simulink model "flightsim_simple_ode_3D_1_5_ListedAssumptions"  (R2020b)
settings: Solver=VariableStepAuto  StartTime=0.0  StopTime=12  RelTol=1e-3
libraries: simulink x3, pid_lib x2
settings Model: Creator=jonathan  LastModifiedBy=jonathan

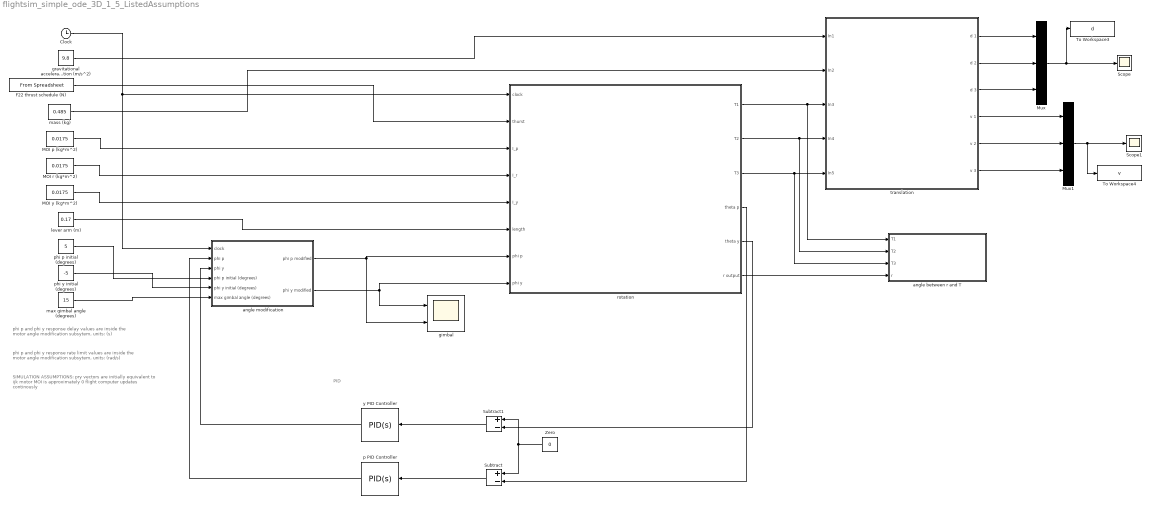
== system flightsim_simple_ode_3D_1_5_ListedAssumptions ==
  note: PID
  note: SIMULATION ASSUMPTIONS:
      | pry vectors are initially equivalent to ijk
      | motor MOI is approximately 0
      | flight computer updates continously
  note: phi p and phi y response rate limit values are inside the motor angle modification subsytem, units: (rad/s)
  note: phi p and phi y response delay values are inside the motor angle modification subsytem, units: (s)
  Clock : Clock
  F22 thrust schedule (N) : FromSpreadsheet  FileName=/Users/jonathan/Documents/GitHub/TVC-6DOF-Flight-Simulation/F15_thrust_curve.xlsx  OutDataTypeStr=double  ExtrapolationBeforeFirstDataPoint=Hold first value  ExtrapolationAfterLastDataPoint=Hold last value
  MOI p (kg*m^2) : Constant  Value=0.0175
  MOI r (kg*m^2) : Constant  Value=0.0175
  MOI y (kg*m^2) : Constant  Value=0.0175
  Mux : Mux  Inputs=3
  Mux1 : Mux  Inputs=3
  Scope : Scope
  Scope1 : Scope
  Subtract : Sum  Inputs=+-
  Subtract1 : Sum  Inputs=+-
  To Workspace3 : ToWorkspace  VariableName=d  SaveFormat=Timeseries  SampleTime=-1
  To Workspace4 : ToWorkspace  VariableName=v  SaveFormat=Timeseries  SampleTime=-1
  Zero : Constant  Value=0  OutDataTypeStr=Inherit: Inherit via back propagation
  angle between r and T : Subsystem
  angle modification : Subsystem
  gimbal : Scope  NumInputPorts=2
  gravitational acceleration (m/s^2) : Constant  Value=9.8
  lever arm (m) : Constant  Value=0.17
  mass (kg) : Constant  Value=0.485
  max gimbal angle (degrees) : Constant  Value=15
  p PID Controller : pid_lib/PID Controller  Controller=PID  Form=Parallel  TimeDomain=Continuous-time  UseExternalTs=off  SampleTime=-1  IntegratorMethod=Forward Euler  FilterMethod=Forward Euler  ControllerParametersSource=internal  P=-0.00942  I=-0.00055  D=-0.03588  UseFilter=on  N=1142.8279760416  TunerSelectOption=Transfer Function Based (PID Tuner App)  InitialConditionSource=internal  InitialConditionForIntegrator=0  InitialConditionForFilter=0  DifferentiatorICPrevScaledInput=0  ExternalReset=none  TrackingMode=off  Kt=1  LimitOutput=off  SatLimitsSource=internal  UpperSaturationLimit=inf  LowerSaturationLimit=-inf  LinearizeAsGain=on  AntiWindupMode=none  Kb=1  POutMin=[]  POutMax=[]  IOutMin=[]  IOutMax=[]  DOutMin=[]  DOutMax=[]  NOutMin=[]  NOutMax=[]  SumOutMin=[]  SumOutMax=[]  SaturationOutMin=[]  SaturationOutMax=[]  PParamMin=[]  PParamMax=[]  IParamMin=[]  IParamMax=[]  DParamMin=[]  DParamMax=[]  NParamMin=[]  NParamMax=[]  KbParamMin=[]  KbParamMax=[]  KtParamMin=[]  KtParamMax=[]  KbOutMin=[]  KbOutMax=[]  KtOutMin=[]  KtOutMax=[]  IntegratorOutMin=[]  IntegratorOutMax=[]  FilterOutMin=[]  FilterOutMax=[]  SumI1OutMin=[]  SumI1OutMax=[]  SumI2OutMin=[]  SumI2OutMax=[]  SumI3OutMin=[]  SumI3OutMax=[]  SumI4OutMin=[]  SumI4OutMax=[]  SumDOutMin=[]  SumDOutMax=[]  DifferentiatorOutMin=[]  DifferentiatorOutMax=[]  FilterDiffOutCoefMin=[]  FilterDiffOutCoefMax=[]  ReciprocalOutMin=[]  ReciprocalOutMax=[]  SumDenOutMin=[]  SumDenOutMax=[]  SumNumOutMin=[]  SumNumOutMax=[]  DivideOutMin=[]  DivideOutMax=[]  UdiffTsProdOutMin=[]  UdiffTsProdOutMax=[]  NTsProdOutMin=[]  NTsProdOutMax=[]  UintegralTsProdOutMin=[]  UintegralTsProdOutMax=[]  UngainTsProdOutMin=[]  UngainTsProdOutMax=[]  IntegratorContinuousStateAttributes=''  IntegratorStateMustResolveToSignalObject=off  IntegratorRTWStateStorageClass=Auto  FilterContinuousStateAttributes=''  FilterStateMustResolveToSignalObject=off  FilterRTWStateStorageClass=Auto  ParallelPVariant=InternalParameters  IdealPVariant=Disabled  IVariant=InternalParameters  DVariant=InternalParameters  IntegratorVariant=Continuous  SatVariant=Disabled  AWVariant=Passthrough  PCopyVariant=Disabled  TRVariant=Disabled  FdbkBlocksVariant=Forward  IdealPFdbkVariant=Disabled  SatFdbkVariant=Disabled  DerivativeFilterVariant=ContFilter  NVariant=InternalParameters  NCopyVariant=Disabled  FilterICVariant=InternalICsFilter  IntegratorICVariant=InternalICs  ExternalResetVariant=Disabled  TRSumVariant=Passthrough  SumFdbkVariant=Disabled  SumVariant=Sum_PID  TsampFilterVariant=InternalTs  TsampNgainVariant=Passthrough  TsampIntegralVariant=Passthrough  ExternalSaturationOutDataTypeStr=Inherit: Same as second input
  phi p initial (degrees) : Constant  Value=5
  phi y initial (degrees) : Constant  Value=-5
  rotation : Subsystem
  translation : Subsystem
  y PID Controller : pid_lib/PID Controller  Controller=PID  Form=Parallel  TimeDomain=Continuous-time  UseExternalTs=off  SampleTime=-1  IntegratorMethod=Forward Euler  FilterMethod=Forward Euler  ControllerParametersSource=internal  P=0.01930  I=0.00113  D=0.07350  UseFilter=on  N=1142.8279760416  TunerSelectOption=Transfer Function Based (PID Tuner App)  InitialConditionSource=internal  InitialConditionForIntegrator=0  InitialConditionForFilter=0  DifferentiatorICPrevScaledInput=0  ExternalReset=none  TrackingMode=off  Kt=1  LimitOutput=off  SatLimitsSource=internal  UpperSaturationLimit=inf  LowerSaturationLimit=-inf  LinearizeAsGain=on  AntiWindupMode=none  Kb=1  POutMin=[]  POutMax=[]  IOutMin=[]  IOutMax=[]  DOutMin=[]  DOutMax=[]  NOutMin=[]  NOutMax=[]  SumOutMin=[]  SumOutMax=[]  SaturationOutMin=[]  SaturationOutMax=[]  PParamMin=[]  PParamMax=[]  IParamMin=[]  IParamMax=[]  DParamMin=[]  DParamMax=[]  NParamMin=[]  NParamMax=[]  KbParamMin=[]  KbParamMax=[]  KtParamMin=[]  KtParamMax=[]  KbOutMin=[]  KbOutMax=[]  KtOutMin=[]  KtOutMax=[]  IntegratorOutMin=[]  IntegratorOutMax=[]  FilterOutMin=[]  FilterOutMax=[]  SumI1OutMin=[]  SumI1OutMax=[]  SumI2OutMin=[]  SumI2OutMax=[]  SumI3OutMin=[]  SumI3OutMax=[]  SumI4OutMin=[]  SumI4OutMax=[]  SumDOutMin=[]  SumDOutMax=[]  DifferentiatorOutMin=[]  DifferentiatorOutMax=[]  FilterDiffOutCoefMin=[]  FilterDiffOutCoefMax=[]  ReciprocalOutMin=[]  ReciprocalOutMax=[]  SumDenOutMin=[]  SumDenOutMax=[]  SumNumOutMin=[]  SumNumOutMax=[]  DivideOutMin=[]  DivideOutMax=[]  UdiffTsProdOutMin=[]  UdiffTsProdOutMax=[]  NTsProdOutMin=[]  NTsProdOutMax=[]  UintegralTsProdOutMin=[]  UintegralTsProdOutMax=[]  UngainTsProdOutMin=[]  UngainTsProdOutMax=[]  IntegratorContinuousStateAttributes=''  IntegratorStateMustResolveToSignalObject=off  IntegratorRTWStateStorageClass=Auto  FilterContinuousStateAttributes=''  FilterStateMustResolveToSignalObject=off  FilterRTWStateStorageClass=Auto  ParallelPVariant=InternalParameters  IdealPVariant=Disabled  IVariant=InternalParameters  DVariant=InternalParameters  IntegratorVariant=Continuous  SatVariant=Disabled  AWVariant=Passthrough  PCopyVariant=Disabled  TRVariant=Disabled  FdbkBlocksVariant=Forward  IdealPFdbkVariant=Disabled  SatFdbkVariant=Disabled  DerivativeFilterVariant=ContFilter  NVariant=InternalParameters  NCopyVariant=Disabled  FilterICVariant=InternalICsFilter  IntegratorICVariant=InternalICs  ExternalResetVariant=Disabled  TRSumVariant=Passthrough  SumFdbkVariant=Disabled  SumVariant=Sum_PID  TsampFilterVariant=InternalTs  TsampNgainVariant=Passthrough  TsampIntegralVariant=Passthrough  ExternalSaturationOutDataTypeStr=Inherit: Same as second input
  wires:
  MOI p (kg*m^2)/1 -> rotation/3(I_p)
  MOI r (kg*m^2)/1 -> rotation/4(I_r)
  MOI y (kg*m^2)/1 -> rotation/5(I_y)
  lever arm (m)/1 -> rotation/6(length)
  rotation/6(r output) -> angle between r and T/4(r)
  gravitational acceleration (m/s^2)/1 -> translation/1(In1)
  mass (kg)/1 -> translation/2(In2)
  rotation/1(T1) -> translation/3(In3), angle between r and T/1(T1)
  rotation/2(T2) -> translation/4(In4), angle between r and T/2(T2)
  rotation/3(T3) -> translation/5(In5), angle between r and T/3(T3)
  translation/4(v 1) -> Mux1/1
  translation/5(v 2) -> Mux1/2
  translation/6(v 3) -> Mux1/3
  translation/1(d 1) -> Mux/1
  translation/2(d 2) -> Mux/2
  translation/3(d 3) -> Mux/3
  Mux/1 -> To Workspace3/1, Scope/1
  Mux1/1 -> Scope1/1, To Workspace4/1
  F22 thrust schedule (N)/1 -> rotation/2(thurst)
  phi y initial (degrees)/1 -> angle modification/5(phi y initial (degrees))
  phi p initial (degrees)/1 -> angle modification/4(phi p initial (degrees))
  Clock/1 -> angle modification/1(clock), rotation/1(clock)
  y PID Controller/1 -> angle modification/3(phi y)
  p PID Controller/1 -> angle modification/2(phi p)
  angle modification/2(phi y modified) -> rotation/8(phi y), gimbal/1
  Zero/1 -> Subtract1/1, Subtract/1
  Subtract1/1 -> y PID Controller/1
  rotation/5(theta y) -> Subtract1/2
  rotation/4(theta p) -> Subtract/2
  angle modification/1(phi p modified) -> rotation/7(phi p), gimbal/2
  max gimbal angle (degrees)/1 -> angle modification/6(max gimbal angle (degrees))
  Subtract/1 -> p PID Controller/1

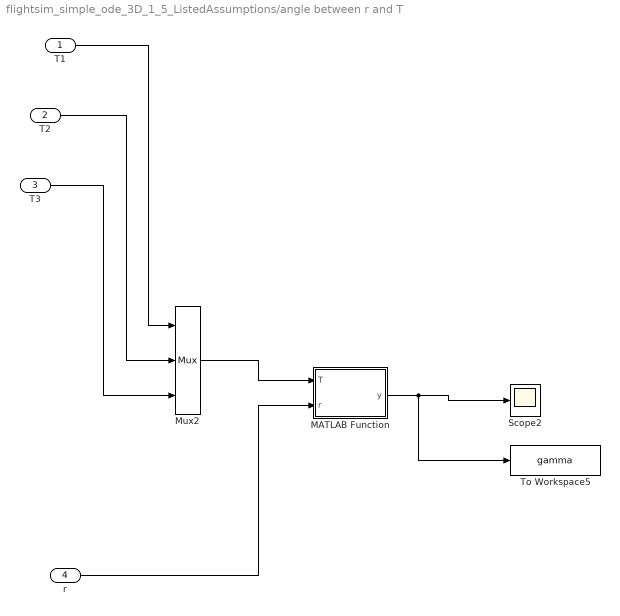
== system flightsim_simple_ode_3D_1_5_ListedAssumptions/angle between r and T ==
  T1 : Inport
  T2 : Inport  Port=2
  T3 : Inport  Port=3
  r : Inport  Port=4
  MATLAB Function : MATLAB Function  TreatAsAtomicUnit=on
  Mux2 : Mux  Inputs=3
  Scope2 : Scope
  To Workspace5 : ToWorkspace  VariableName=gamma  SaveFormat=Timeseries  SampleTime=-1
  wires:
  T3/1 -> Mux2/3
  r/1 -> MATLAB Function/2(r)
  T2/1 -> Mux2/2
  T1/1 -> Mux2/1
  Mux2/1 -> MATLAB Function/1(T)
  MATLAB Function/1(y) -> To Workspace5/1, Scope2/1

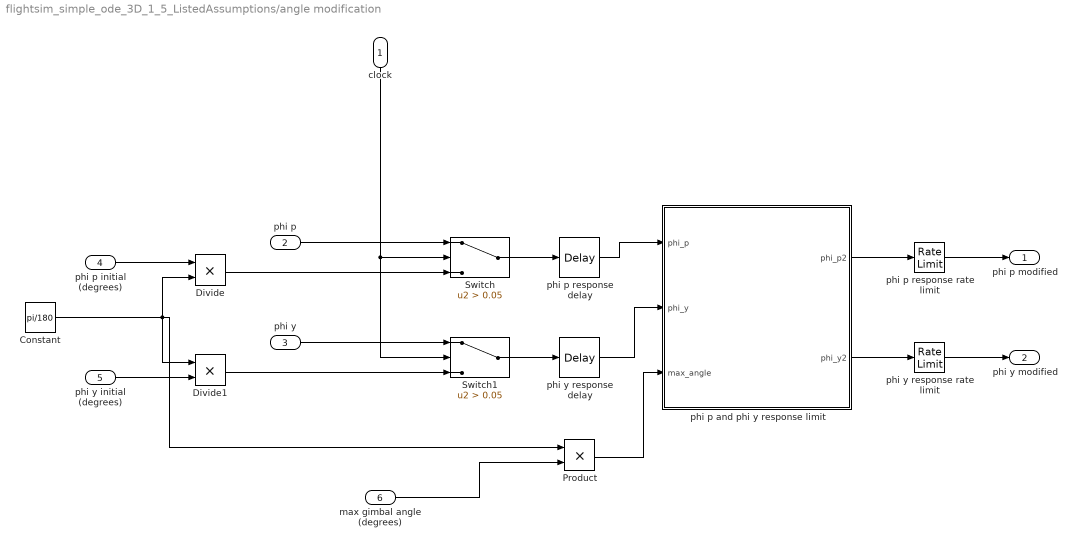
== system flightsim_simple_ode_3D_1_5_ListedAssumptions/angle modification ==
  clock : Inport
  phi p : Inport  Port=2
  phi y : Inport  Port=3
  phi p initial (degrees) : Inport  Port=4
  phi y initial (degrees) : Inport  Port=5
  max gimbal angle (degrees) : Inport  Port=6
  Constant : Constant  Value=pi/180
  Divide : Product  Inputs=**
  Divide1 : Product  Inputs=**
  Product : Product
  Switch : Switch  Criteria=u2 > Threshold  Threshold=0.05
  Switch1 : Switch  Criteria=u2 > Threshold  Threshold=0.05
  phi p and phi y response limit : MATLAB Function  TreatAsAtomicUnit=on
  phi p response delay : TransportDelay  DelayTime=0.05
  phi p response rate limit : RateLimiter  RisingSlewLimit=175*pi/180  FallingSlewLimit=-175*pi/180  SampleTimeMode=inherited
  phi y response delay : TransportDelay  DelayTime=0.05
  phi y response rate limit : RateLimiter  RisingSlewLimit=175*pi/180  FallingSlewLimit=-175*pi/180  SampleTimeMode=inherited
  phi p modified : Outport
  phi y modified : Outport  Port=2
  wires:
  phi p/1 -> Switch/1
  phi y/1 -> Switch1/1
  clock/1 -> Switch/2, Switch1/2
  phi p initial (degrees)/1 -> Divide/1
  Constant/1 -> Product/1, Divide1/1, Divide/2
  Divide/1 -> Switch/3
  Divide1/1 -> Switch1/3
  phi y initial (degrees)/1 -> Divide1/2
  Switch1/1 -> phi y response delay/1
  phi p response rate limit/1 -> phi p modified/1
  phi y response rate limit/1 -> phi y modified/1
  Switch/1 -> phi p response delay/1
  phi p response delay/1 -> phi p and phi y response limit/1(phi_p)
  phi y response delay/1 -> phi p and phi y response limit/2(phi_y)
  phi p and phi y response limit/1(phi_p2) -> phi p response rate limit/1
  phi p and phi y response limit/2(phi_y2) -> phi y response rate limit/1
  max gimbal angle (degrees)/1 -> Product/2
  Product/1 -> phi p and phi y response limit/3(max_angle)

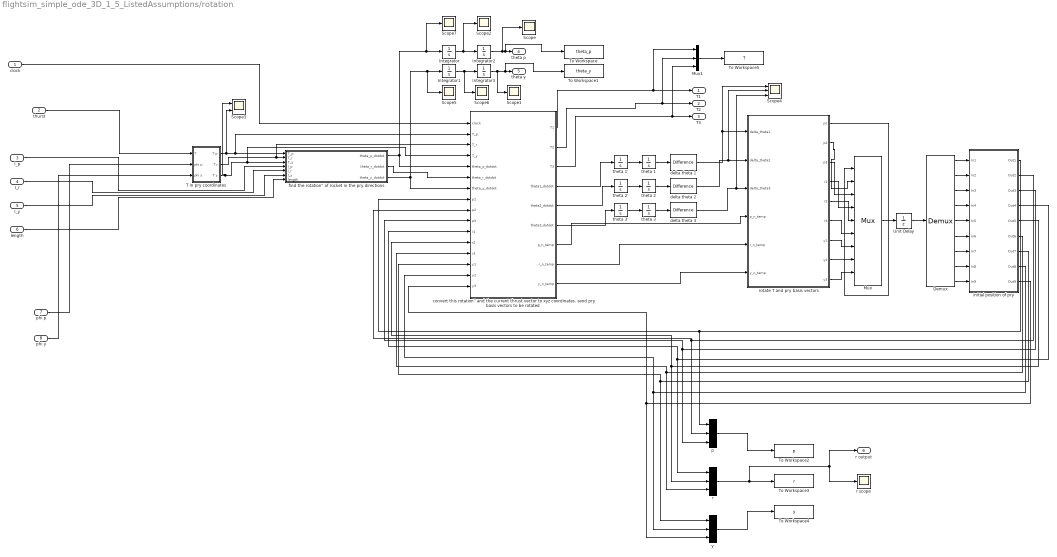
== system flightsim_simple_ode_3D_1_5_ListedAssumptions/rotation ==
  clock : Inport
  thurst : Inport  Port=2
  I_p : Inport  Port=3
  I_r : Inport  Port=4
  I_y : Inport  Port=5
  length : Inport  Port=6
  phi p : Inport  Port=7
  phi y : Inport  Port=8
  Demux : Demux  Outputs=9
  Integrator{,1..3} (4 alike) : Integrator
  Mux : Mux  Inputs=9
  Mux1 : Mux  Inputs=3
  Scope{,1..2,5..7} (6 alike) : Scope
  Scope3 : Scope  NumInputPorts=2
  Scope4 : Scope  NumInputPorts=3
  T in pry coordinates : Subsystem
  To Workspace : ToWorkspace  VariableName=theta_p  SaveFormat=Timeseries  SampleTime=-1
  To Workspace1 : ToWorkspace  VariableName=theta_y  SaveFormat=Timeseries  SampleTime=-1
  To Workspace2 : ToWorkspace  VariableName=p  SaveFormat=Timeseries  SampleTime=-1
  To Workspace3 : ToWorkspace  VariableName=r  SaveFormat=Timeseries  SampleTime=-1
  To Workspace4 : ToWorkspace  VariableName=y  SaveFormat=Timeseries  SampleTime=-1
  To Workspace5 : ToWorkspace  VariableName=T  SaveFormat=Timeseries  SampleTime=-1
  Unit Delay : UnitDelay  SampleTime=0.05  HasFrameUpgradeWarning=on
  convert this rotation'' and the current thrust vector to xyz coordinates. send pry basis vectors to be rotated : MATLAB Function  TreatAsAtomicUnit=on
  delta theta 1 : simulink/Quick Insert/Discrete/Difference  ICPrevInput=0.0  OutMin=[]  OutMax=[]  OutDataType=fixdt(1, 16)  OutScaling=2^-10  DoSatur=off
      settings: SourceProductBaseCode=SL
  delta theta 2 : simulink/Quick Insert/Discrete/Difference  ICPrevInput=0.0  OutMin=[]  OutMax=[]  OutDataType=fixdt(1, 16)  OutScaling=2^-10  DoSatur=off
      settings: SourceProductBaseCode=SL
  delta theta 3 : simulink/Quick Insert/Discrete/Difference  ICPrevInput=0.0  OutMin=[]  OutMax=[]  OutDataType=fixdt(1, 16)  OutScaling=2^-10  DoSatur=off
      settings: SourceProductBaseCode=SL
  find the rotation'' of rocket in the pry directions : MATLAB Function  TreatAsAtomicUnit=on
  initial position of pry : Subsystem
  p : Mux  Inputs=3
  r : Mux  Inputs=3
  r scope : Scope
  rotate T and pry basis vectors : MATLAB Function  TreatAsAtomicUnit=on
  theta 1 : Integrator
  theta 1' : Integrator
  theta 2 : Integrator
  theta 2' : Integrator
  theta 3 : Integrator
  theta 3' : Integrator
  y : Mux  Inputs=3
  T1 : Outport
  T2 : Outport  Port=2
  T3 : Outport  Port=3
  theta p : Outport  Port=4
  theta y : Outport  Port=5
  r output : Outport  Port=6
  wires:
  length/1 -> find the rotation'' of rocket in the pry directions/7(length)
  y/1 -> To Workspace4/1
  convert this rotation'' and the current thrust vector to xyz coordinates. send pry basis vectors to be rotated/9(y_n_temp) -> rotate T and pry basis vectors/6(y_n_temp)
  T in pry coordinates/1(T p) -> Scope3/2, convert this rotation'' and the current thrust vector to xyz coordinates. send pry basis vectors to be rotated/2(T_p), find the rotation'' of rocket in the pry directions/1(T_p)
  clock/1 -> convert this rotation'' and the current thrust vector to xyz coordinates. send pry basis vectors to be rotated/1(clock)
  theta 2'/1 -> theta 2/1
  theta 1'/1 -> theta 1/1
  theta 3'/1 -> theta 3/1
  convert this rotation'' and the current thrust vector to xyz coordinates. send pry basis vectors to be rotated/8(r_n_temp) -> rotate T and pry basis vectors/5(r_n_temp)
  find the rotation'' of rocket in the pry directions/2(theta_r_dotdot) -> convert this rotation'' and the current thrust vector to xyz coordinates. send pry basis vectors to be rotated/6(theta_r_dotdot)
  T in pry coordinates/2(T r) -> convert this rotation'' and the current thrust vector to xyz coordinates. send pry basis vectors to be rotated/3(T_r), find the rotation'' of rocket in the pry directions/2(T_r)
  theta 2/1 -> delta theta 2/1
  convert this rotation'' and the current thrust vector to xyz coordinates. send pry basis vectors to be rotated/3(T3) -> Mux1/3, T3/1
  r/1 -> r scope/1, r output/1, To Workspace3/1
  phi y/1 -> T in pry coordinates/3(phi y)
  convert this rotation'' and the current thrust vector to xyz coordinates. send pry basis vectors to be rotated/7(p_n_temp) -> rotate T and pry basis vectors/4(p_n_temp)
  phi p/1 -> T in pry coordinates/2(phi p)
  convert this rotation'' and the current thrust vector to xyz coordinates. send pry basis vectors to be rotated/2(T2) -> Mux1/2, T2/1
  p/1 -> To Workspace2/1
  convert this rotation'' and the current thrust vector to xyz coordinates. send pry basis vectors to be rotated/6(theta3_dotdot) -> theta 3'/1
  I_r/1 -> find the rotation'' of rocket in the pry directions/5(I_r)
  convert this rotation'' and the current thrust vector to xyz coordinates. send pry basis vectors to be rotated/1(T1) -> Mux1/1, T1/1
  convert this rotation'' and the current thrust vector to xyz coordinates. send pry basis vectors to be rotated/5(theta2_dotdot) -> theta 2'/1
  convert this rotation'' and the current thrust vector to xyz coordinates. send pry basis vectors to be rotated/4(theta1_dotdot) -> theta 1'/1
  thurst/1 -> T in pry coordinates/1(T)
  I_p/1 -> find the rotation'' of rocket in the pry directions/4(I_p)
  I_y/1 -> find the rotation'' of rocket in the pry directions/6(I_y)
  Integrator/1 -> Scope2/1, Integrator2/1
  find the rotation'' of rocket in the pry directions/1(theta_p_dotdot) -> convert this rotation'' and the current thrust vector to xyz coordinates. send pry basis vectors to be rotated/5(theta_p_dotdot), Scope7/1, Integrator/1
  find the rotation'' of rocket in the pry directions/3(theta_y_dotdot) -> convert this rotation'' and the current thrust vector to xyz coordinates. send pry basis vectors to be rotated/7(theta_y_dotdot), Scope5/1, Integrator1/1
  Integrator2/1 -> Scope/1, To Workspace/1, theta p/1
  Integrator3/1 -> Scope1/1, To Workspace1/1, theta y/1
  theta 3/1 -> delta theta 3/1
  rotate T and pry basis vectors/1(p1) -> Mux/1
  rotate T and pry basis vectors/2(p2) -> Mux/2
  rotate T and pry basis vectors/3(p3) -> Mux/3
  rotate T and pry basis vectors/4(r1) -> Mux/4
  rotate T and pry basis vectors/5(r2) -> Mux/5
  rotate T and pry basis vectors/6(r3) -> Mux/6
  rotate T and pry basis vectors/7(y1) -> Mux/7
  rotate T and pry basis vectors/8(y2) -> Mux/8
  rotate T and pry basis vectors/9(y3) -> Mux/9
  initial position of pry/7(Out7) -> y/1, convert this rotation'' and the current thrust vector to xyz coordinates. send pry basis vectors to be rotated/14(y1)
  initial position of pry/8(Out8) -> y/2, convert this rotation'' and the current thrust vector to xyz coordinates. send pry basis vectors to be rotated/15(y2)
  initial position of pry/4(Out4) -> r/1, convert this rotation'' and the current thrust vector to xyz coordinates. send pry basis vectors to be rotated/11(r1)
  initial position of pry/5(Out5) -> r/2, convert this rotation'' and the current thrust vector to xyz coordinates. send pry basis vectors to be rotated/12(r2)
  initial position of pry/6(Out6) -> r/3, convert this rotation'' and the current thrust vector to xyz coordinates. send pry basis vectors to be rotated/13(r3)
  initial position of pry/1(Out1) -> p/1, convert this rotation'' and the current thrust vector to xyz coordinates. send pry basis vectors to be rotated/8(p1)
  initial position of pry/9(Out9) -> y/3, convert this rotation'' and the current thrust vector to xyz coordinates. send pry basis vectors to be rotated/16(y3)
  initial position of pry/3(Out3) -> p/3, convert this rotation'' and the current thrust vector to xyz coordinates. send pry basis vectors to be rotated/10(p3)
  initial position of pry/2(Out2) -> p/2, convert this rotation'' and the current thrust vector to xyz coordinates. send pry basis vectors to be rotated/9(p2)
  Demux/1 -> initial position of pry/1(In1)
  Demux/2 -> initial position of pry/2(In2)
  Demux/3 -> initial position of pry/3(In3)
  Demux/4 -> initial position of pry/4(In4)
  Demux/5 -> initial position of pry/5(In5)
  Demux/6 -> initial position of pry/6(In6)
  Demux/7 -> initial position of pry/7(In7)
  Demux/8 -> initial position of pry/8(In8)
  Demux/9 -> initial position of pry/9(In9)
  T in pry coordinates/3(T y) -> Scope3/1, convert this rotation'' and the current thrust vector to xyz coordinates. send pry basis vectors to be rotated/4(T_y), find the rotation'' of rocket in the pry directions/3(T_y)
  Mux1/1 -> To Workspace5/1
  theta 1/1 -> delta theta 1/1
  delta theta 1/1 -> Scope4/1, rotate T and pry basis vectors/1(delta_theta1)
  delta theta 2/1 -> Scope4/2, rotate T and pry basis vectors/2(delta_theta2)
  delta theta 3/1 -> Scope4/3, rotate T and pry basis vectors/3(delta_theta3)
  Integrator1/1 -> Scope6/1, Integrator3/1
  Mux/1 -> Unit Delay/1
  Unit Delay/1 -> Demux/1

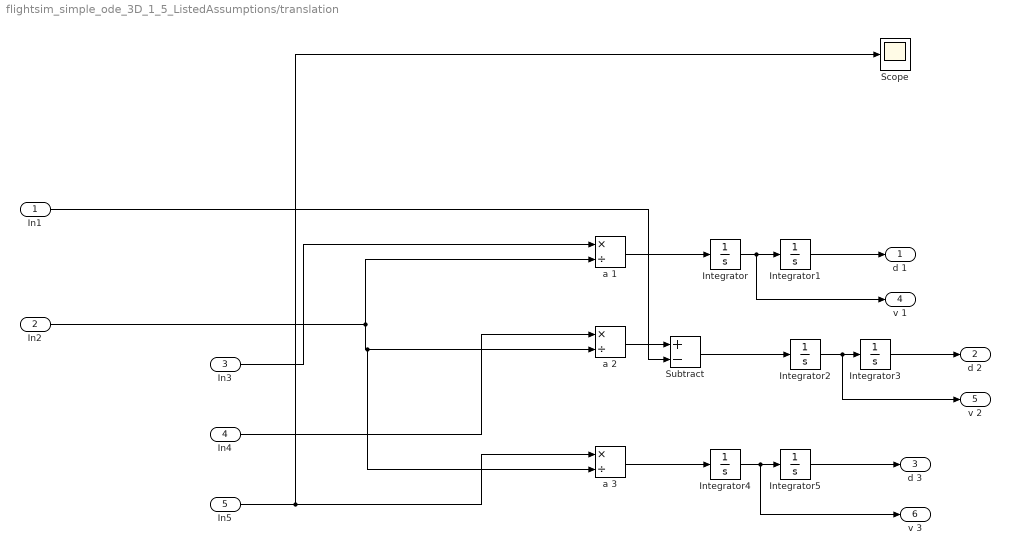
== system flightsim_simple_ode_3D_1_5_ListedAssumptions/translation ==
  In1 : Inport
  In2 : Inport  Port=2
  In3 : Inport  Port=3
  In4 : Inport  Port=4
  In5 : Inport  Port=5
  Integrator{,1..5} (6 alike) : Integrator
  Scope : Scope
  Subtract : Sum  Inputs=+-
  a 1 : Product  Inputs=*/
  a 2 : Product  Inputs=*/
  a 3 : Product  Inputs=*/
  d 1 : Outport
  d 2 : Outport  Port=2
  d 3 : Outport  Port=3
  v 1 : Outport  Port=4
  v 2 : Outport  Port=5
  v 3 : Outport  Port=6
  wires:
  Integrator5/1 -> d 3/1
  In4/1 -> a 2/1
  In5/1 -> Scope/1, a 3/1
  In3/1 -> a 1/1
  Subtract/1 -> Integrator2/1
  a 2/1 -> Subtract/1
  In1/1 -> Subtract/2
  In2/1 -> a 3/2, a 2/2, a 1/2
  Integrator/1 -> v 1/1, Integrator1/1
  a 1/1 -> Integrator/1
  Integrator2/1 -> v 2/1, Integrator3/1
  a 3/1 -> Integrator4/1
  Integrator4/1 -> v 3/1, Integrator5/1
  Integrator1/1 -> d 1/1
  Integrator3/1 -> d 2/1

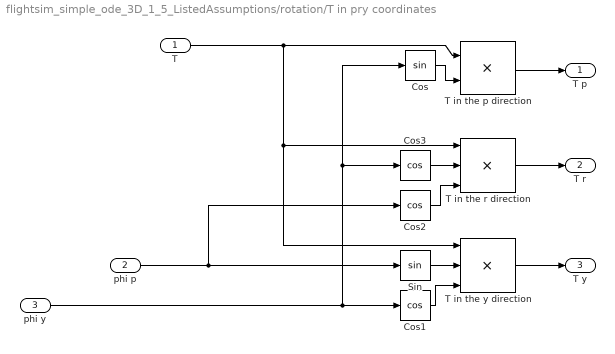
== system flightsim_simple_ode_3D_1_5_ListedAssumptions/rotation/T in pry coordinates ==
  T : Inport
  phi p : Inport  Port=2
  phi y : Inport  Port=3
  Cos : Trigonometry
  Cos1 : Trigonometry  Operator=cos
  Cos2 : Trigonometry  Operator=cos
  Cos3 : Trigonometry  Operator=cos
  Sin : Trigonometry
  T in the p direction : Product  Inputs=**
  T in the r direction : Product  Inputs=***
  T in the y direction : Product  Inputs=***
  T p : Outport
  T r : Outport  Port=2
  T y : Outport  Port=3
  wires:
  Cos3/1 -> T in the r direction/2
  Cos1/1 -> T in the y direction/3
  Cos/1 -> T in the p direction/2
  T in the p direction/1 -> T p/1
  T/1 -> T in the y direction/1, T in the r direction/1, T in the p direction/1
  Sin/1 -> T in the y direction/2
  Cos2/1 -> T in the r direction/3
  T in the y direction/1 -> T y/1
  phi p/1 -> Cos2/1, Sin/1
  phi y/1 -> Cos/1, Cos3/1, Cos1/1
  T in the r direction/1 -> T r/1

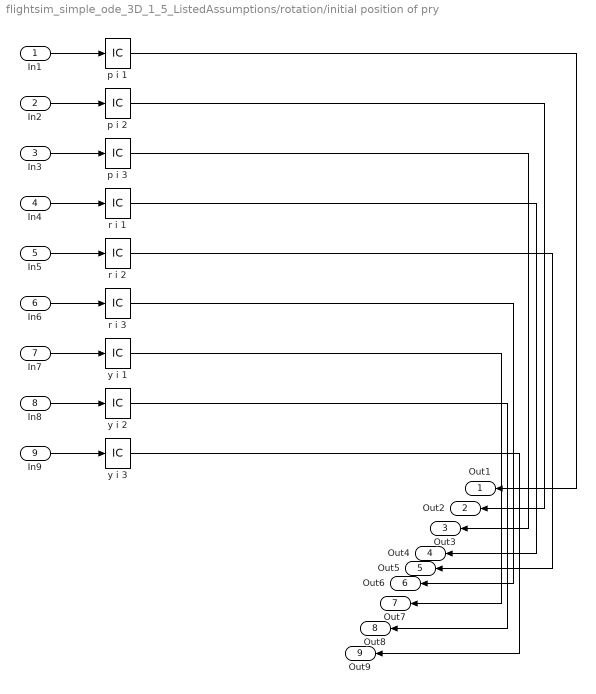
== system flightsim_simple_ode_3D_1_5_ListedAssumptions/rotation/initial position of pry ==
  In1 : Inport
  In2 : Inport  Port=2
  In3 : Inport  Port=3
  In4 : Inport  Port=4
  In5 : Inport  Port=5
  In6 : Inport  Port=6
  In7 : Inport  Port=7
  In8 : Inport  Port=8
  In9 : Inport  Port=9
  p i 1 : InitialCondition
  p i 2 : InitialCondition  Value=0
  p i 3 : InitialCondition  Value=0
  r i 1 : InitialCondition  Value=0
  r i 2 : InitialCondition
  r i 3 : InitialCondition  Value=0
  y i 1 : InitialCondition  Value=0
  y i 2 : InitialCondition  Value=0
  y i 3 : InitialCondition
  Out1 : Outport
  Out2 : Outport  Port=2
  Out3 : Outport  Port=3
  Out4 : Outport  Port=4
  Out5 : Outport  Port=5
  Out6 : Outport  Port=6
  Out7 : Outport  Port=7
  Out8 : Outport  Port=8
  Out9 : Outport  Port=9
  wires:
  p i 2/1 -> Out2/1
  y i 1/1 -> Out7/1
  In3/1 -> p i 3/1
  r i 2/1 -> Out5/1
  r i 1/1 -> Out4/1
  y i 2/1 -> Out8/1
  In5/1 -> r i 2/1
  r i 3/1 -> Out6/1
  In9/1 -> y i 3/1
  p i 1/1 -> Out1/1
  In2/1 -> p i 2/1
  In4/1 -> r i 1/1
  In8/1 -> y i 2/1
  p i 3/1 -> Out3/1
  In7/1 -> y i 1/1
  In1/1 -> p i 1/1
  y i 3/1 -> Out9/1
  In6/1 -> r i 3/1

== matlab function flightsim_simple_ode_3D_1_5_ListedAssumptions/angle between r and T/MATLAB Function ==
  data: T input; y output; r input
function y = fcn(T,r)

U = T;
V = r;

y = acos(dot(U,V)/(norm(U)*norm(V)));

== matlab function flightsim_simple_ode_3D_1_5_ListedAssumptions/angle modification/phi p and phi y response limit ==
  data: phi_p input; phi_p2 output; phi_y input; phi_y2 output; max_angle input
function [phi_p2, phi_y2] = fcn(phi_p, phi_y, max_angle)

% max_angle - maximum angle that motor can tilt from vertical axis

sigma = atan(sin(phi_p)/tan(phi_y)); % sets direction of thrust

phi_p2 = phi_p;
phi_y2 = phi_y;

while (asin(sqrt( (sin(phi_y2)^2) + ((sin(phi_p2)*cos(phi_y2))^2) )) > max_angle)
    if (phi_p2 > 0)
        phi_p2 = phi_p2 - 0.01;
    else
        phi_p2 = phi_p2 + 0.01;
    end
    
    phi_y2 = atan(sin(phi_p2)/tan(sigma));
end

== matlab function flightsim_simple_ode_3D_1_5_ListedAssumptions/rotation/convert this rotation'' and the current thrust vector to xyz coordinates. send pry basis vectors to be rotated ==
  data: T1 output; T2 output; T3 output; clock input; T_p input; T_r input; T_y input; theta_p_dotdot input; theta1_dotdot output; theta_r_dotdot input; theta_y_dotdot input; p1 input; p2 input; p3 input; theta2_dotdot output; theta3_dotdot output; p_n_temp output; r_n_temp output; y_n_temp output; r1 input; r2 input; r3 input; y1 input; y2 input; y3 input
function [T1, T2, T3, theta1_dotdot, theta2_dotdot, theta3_dotdot, p_n_temp, r_n_temp, y_n_temp] = fcn(clock, T_p, T_r, T_y, theta_p_dotdot, theta_r_dotdot, theta_y_dotdot, p1, p2, p3, r1, r2, r3, y1, y2, y3)

% if clock == 0
%     B = [p_i, r_i, y_i];
%     
%     p_n_temp = p_i;
%     r_n_temp = r_i;
%     y_n_temp = y_i;
% else
    p = [p1; p2; p3];
    r = [r1; r2; r3];
    y = [y1; y2; y3];
    
    B = [p, r, y];
    
    p_n_temp = p;
    r_n_temp = r;
    y_n_temp = y;
% end

% covert T from pry to ijk
v = B*[T_p; T_r; T_y];
T1 = v(1);
T2 = v(2);
T3 = v(3);

% covert theta'' from pry to ijk
v = B*[theta_p_dotdot; theta_r_dotdot; theta_y_dotdot];
theta1_dotdot = v(1);
theta2_dotdot = v(2); 
theta3_dotdot = v(3);

== matlab function flightsim_simple_ode_3D_1_5_ListedAssumptions/rotation/find the rotation'' of rocket in the pry directions ==
  data: T_p input; theta_p_dotdot output; T_r input; T_y input; I_p input; I_r input; I_y input; theta_r_dotdot output; theta_y_dotdot output; length input
function [theta_p_dotdot, theta_r_dotdot, theta_y_dotdot] = fcn(T_p,T_r,T_y,I_p,I_r,I_y,length)

C = cross([0, -length, 0], [T_p,T_r,T_y]);
theta_p_dotdot = C(1);
theta_r_dotdot = C(2);
theta_y_dotdot = C(3);

theta_p_dotdot = theta_p_dotdot/I_p;
theta_r_dotdot = theta_r_dotdot/I_r;
theta_y_dotdot = theta_y_dotdot/I_y;

== matlab function flightsim_simple_ode_3D_1_5_ListedAssumptions/rotation/rotate T and pry basis vectors ==
  data: p1 output; p2 output; p3 output; delta_theta1 input; delta_theta2 input; delta_theta3 input; p_n_temp input; r_n_temp input; y_n_temp input; r1 output; r2 output; r3 output; y1 output; y2 output; y3 output
function [p1, p2, p3, r1, r2, r3, y1, y2, y3] = fcn(delta_theta1, delta_theta2, delta_theta3, p_n_temp, r_n_temp, y_n_temp)

R = [cos(delta_theta3), -sin(delta_theta3), 0;
     sin(delta_theta3),  cos(delta_theta3), 0;
          0,       0, 1];
       
R = R*[cos(delta_theta2), 0, sin(delta_theta2);
            0, 1,      0;
      -sin(delta_theta2), 0, cos(delta_theta2)];
  
R = R*[1,      0,       0;
       0, cos(delta_theta1), -sin(delta_theta1);
       0, sin(delta_theta1),  cos(delta_theta1)];


v = R*p_n_temp;
p1 = v(1);
p2 = v(2);
p3 = v(3);

v = R*r_n_temp;
r1 = v(1);
r2 = v(2);
r3 = v(3);

v = R*y_n_temp;
y1 = v(1);
y2 = v(2);
y3 = v(3);
